simulink model "MPC_framework"  (Simulink 7.9)
settings: Solver=FixedStepDiscrete  StartTime=0.0  StopTime=10.0  FixedStep=0.01  RelTol=1e-3
PreLoadFcn:
  | RTWConfigurationCB('preloadfcn', bdroot);
InitFcn:
  | % START RTW CONFIGURATION CODE %
  | RTWConfigurationCB('rtw_target_initfcn',gcs);
  | % END RTW CONFIGURATION CODE %
libraries: mpc5xxobsoleteblocks x13, canblocks x12, simulink x2
settings Model: Creator=Bazs  LastModifiedBy=Bazs
settings OptimizationCC: InitFltsAndDblsToZero=on
settings DebuggingCC: SaveWithParameterizedLinksMsg=none  SignalResolutionControl=TryResolveAllWithWarning  MultiTaskDSMMsg=warning  MultiTaskCondExecSysMsg=none  FcnCallInpInsideContextMsg=Use local settings  StrictBusMsg=Warning
settings SFSimCC: SimParseCustomCode=off
settings RTWCC: IncludeERTFirstTime=on
settings GRTTargetCC: TargetFcnLib=ansi_tfl_tmw.mat  CombineOutputUpdateFcns=off  GRTInterface=on

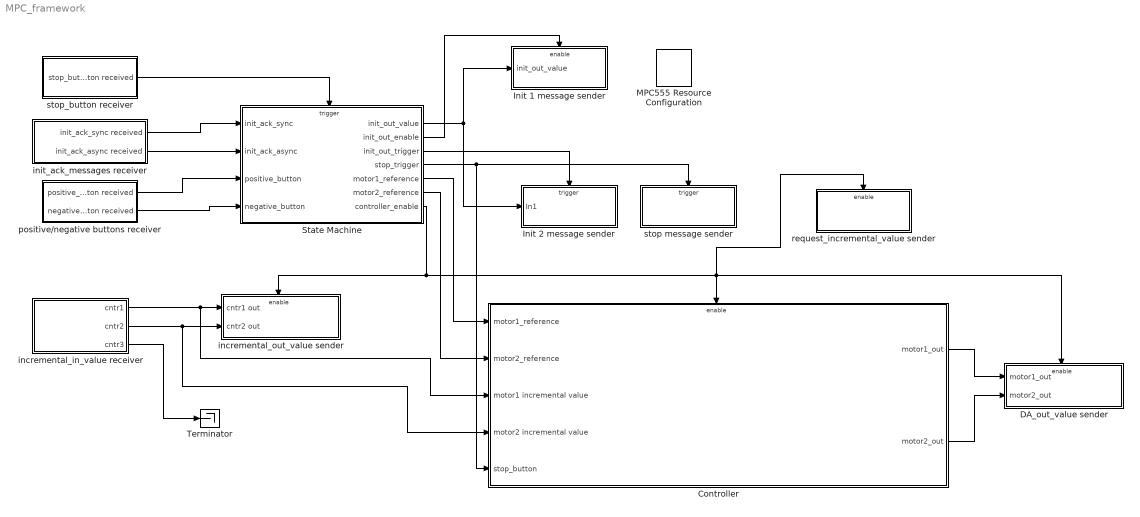
== system MPC_framework ==
  Controller : Subsystem
  DA_out_value sender : Subsystem  TreatAsAtomicUnit=on
  Init 1 message sender : Subsystem  TreatAsAtomicUnit=on
  Init 2 message sender : Subsystem  TreatAsAtomicUnit=on
  MPC555 Resource Configuration : mpc5xxobsoleteblocks/MPC555 Resource Configuration  Tag=RTW CONFIGURATION BLOCK  Priority=-100000  oldParentName=MPC_framework  oldBlockName=|
      | MPC_framework/MPC555
      | Resource
      | Configuration
  State Machine : Stateflow chart  TreatAsAtomicUnit=on
  Terminator : Terminator
  incremental_in_value receiver : Subsystem
  incremental_out_value sender : Subsystem  TreatAsAtomicUnit=on
  init_ack_messages receiver : Subsystem
  positive/negative buttons receiver : Subsystem
  request_incremental_value sender : Subsystem  TreatAsAtomicUnit=on
  stop message sender : Subsystem  TreatAsAtomicUnit=on
  stop_button receiver : Subsystem
  wires:
  State Machine/1(init_out_value) -> Init 1 message sender/1(init_out_value), Init 2 message sender/1(In1)
  State Machine/2(init_out_enable) -> Init 1 message sender/Enable
  init_ack_messages receiver/1(init_ack_sync received) -> State Machine/1(init_ack_sync)
  init_ack_messages receiver/2(init_ack_async received) -> State Machine/2(init_ack_async)
  State Machine/3(init_out_trigger) -> Init 2 message sender/Trigger
  stop_button receiver/1(stop_button received) -> State Machine/Trigger
  State Machine/4(stop_trigger) -> stop message sender/Trigger, Controller/5(stop_button)
  positive/negative buttons receiver/1(positive_button received) -> State Machine/3(positive_button)
  positive/negative buttons receiver/2(negative_button received) -> State Machine/4(negative_button)
  State Machine/7(controller_enable) -> Controller/Enable, DA_out_value sender/Enable, request_incremental_value sender/Enable, incremental_out_value sender/Enable
  State Machine/5(motor1_reference) -> Controller/1(motor1_reference)
  State Machine/6(motor2_reference) -> Controller/2(motor2_reference)
  Controller/1(motor1_out) -> DA_out_value sender/1(motor1_out)
  Controller/2(motor2_out) -> DA_out_value sender/2(motor2_out)
  incremental_in_value receiver/1(cntr1) -> incremental_out_value sender/1(cntr1 out), Controller/3(motor1 incremental value)
  incremental_in_value receiver/2(cntr2) -> incremental_out_value sender/2(cntr2 out), Controller/4(motor2 incremental value)
  incremental_in_value receiver/3(cntr3) -> Terminator/1

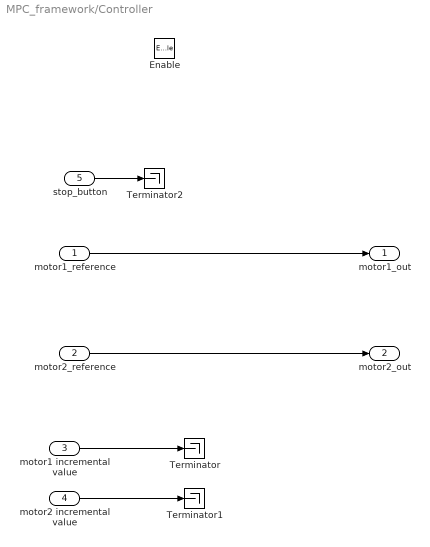
== system MPC_framework/Controller ==
  motor1_reference : Inport
  motor2_reference : Inport  Port=2
  motor1 incremental value : Inport  Port=3
  motor2 incremental value : Inport  Port=4
  stop_button : Inport  Port=5
  Enable : EnablePort
  Terminator : Terminator
  Terminator1 : Terminator
  Terminator2 : Terminator
  motor1_out : Outport
  motor2_out : Outport  Port=2
  wires:
  motor1 incremental value/1 -> Terminator/1
  motor2 incremental value/1 -> Terminator1/1
  motor1_reference/1 -> motor1_out/1
  motor2_reference/1 -> motor2_out/1
  stop_button/1 -> Terminator2/1

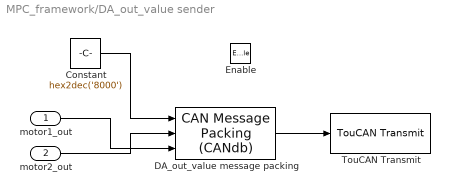
== system MPC_framework/DA_out_value sender ==
  motor1_out : Inport
  motor2_out : Inport  Port=2
  Enable : EnablePort
  Constant : Constant  Value=hex2dec('8000')
  DA_out_value message packing : canblocks/CAN Message Packing (CANdb)
  TouCAN Transmit : mpc5xxobsoleteblocks/CAN 2.0B Controller Module/TouCAN Transmit  module=A  tx_mode=Queued transmission with shared buffer  fifo_queue_length=8  bufferids=0  buffers_used=0, 1, 2  t=-1  enablePassThru=off
  wires:
  DA_out_value message packing/1 -> TouCAN Transmit/1
  motor1_out/1 -> DA_out_value message packing/3
  motor2_out/1 -> DA_out_value message packing/2
  Constant/1 -> DA_out_value message packing/1

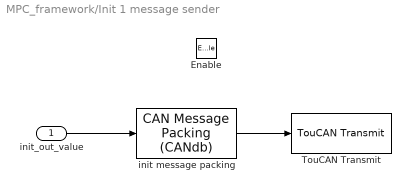
== system MPC_framework/Init 1 message sender ==
  init_out_value : Inport
  Enable : EnablePort
  TouCAN Transmit : mpc5xxobsoleteblocks/CAN 2.0B Controller Module/TouCAN Transmit  module=A  tx_mode=Queued transmission with shared buffer  fifo_queue_length=8  bufferids=0  buffers_used=0, 1, 2  t=-1  enablePassThru=off
  init message packing : canblocks/CAN Message Packing (CANdb)
  wires:
  init_out_value/1 -> init message packing/1
  init message packing/1 -> TouCAN Transmit/1

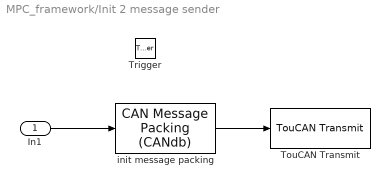
== system MPC_framework/Init 2 message sender ==
  In1 : Inport
  Trigger : TriggerPort
  TouCAN Transmit : mpc5xxobsoleteblocks/CAN 2.0B Controller Module/TouCAN Transmit  module=A  tx_mode=Queued transmission with shared buffer  fifo_queue_length=8  bufferids=0  buffers_used=0, 1, 2  t=-1  enablePassThru=off
  init message packing : canblocks/CAN Message Packing (CANdb)
  wires:
  In1/1 -> init message packing/1
  init message packing/1 -> TouCAN Transmit/1

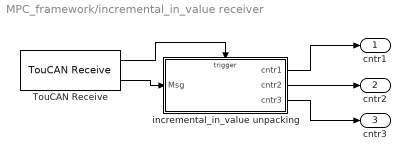
== system MPC_framework/incremental_in_value receiver ==
  TouCAN Receive : mpc5xxobsoleteblocks/CAN 2.0B Controller Module/TouCAN Receive  module=A  ids=hex2dec('07')  message_type=Standard (11-bit identifier)  notification_type=Function Call Outport  auto_select_buffer=on  bufferids=3  use_queue=off  queue_length=3  can_msg=Use unpacking block  t=-1
  incremental_in_value unpacking : Subsystem  TreatAsAtomicUnit=on
      settings: OpenFcn=open_system(gcb, 'force');
      mask Type: CAN Message Unpacking (CANdb)
      mask Description: CAN Message Unpacking (CANdb) Function-Call Subsystem Template
      mask Help: helpview([docroot '/toolbox/can_blocks/can_blocks.map'], 'template_CANdb_msg_unpack');
  cntr1 : Outport
  cntr2 : Outport  Port=2
  cntr3 : Outport  Port=3
  wires:
  incremental_in_value unpacking/1(cntr1) -> cntr1/1
  TouCAN Receive/2 -> incremental_in_value unpacking/1(Msg)
  TouCAN Receive/1 -> incremental_in_value unpacking/Trigger
  incremental_in_value unpacking/2(cntr2) -> cntr2/1
  incremental_in_value unpacking/3(cntr3) -> cntr3/1

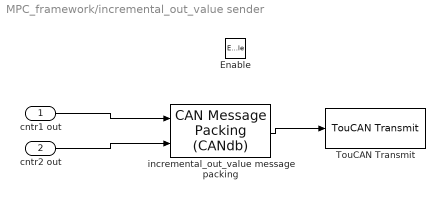
== system MPC_framework/incremental_out_value sender ==
  cntr1 out : Inport
  cntr2 out : Inport  Port=2
  Enable : EnablePort
  TouCAN Transmit : mpc5xxobsoleteblocks/CAN 2.0B Controller Module/TouCAN Transmit  module=A  tx_mode=Queued transmission with shared buffer  fifo_queue_length=8  bufferids=0  buffers_used=0, 1, 2  t=-1  enablePassThru=off
  incremental_out_value message packing : canblocks/CAN Message Packing (CANdb)
  wires:
  incremental_out_value message packing/1 -> TouCAN Transmit/1
  cntr1 out/1 -> incremental_out_value message packing/1
  cntr2 out/1 -> incremental_out_value message packing/2

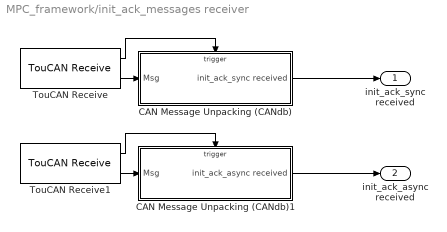
== system MPC_framework/init_ack_messages receiver ==
  CAN Message Unpacking (CANdb) : Subsystem  TreatAsAtomicUnit=on
      settings: OpenFcn=open_system(gcb, 'force');
      mask Type: CAN Message Unpacking (CANdb)
      mask Description: CAN Message Unpacking (CANdb) Function-Call Subsystem Template
      mask Help: helpview([docroot '/toolbox/can_blocks/can_blocks.map'], 'template_CANdb_msg_unpack');
  CAN Message Unpacking (CANdb)1 : Subsystem  TreatAsAtomicUnit=on
      settings: OpenFcn=open_system(gcb, 'force');
      mask Type: CAN Message Unpacking (CANdb)
      mask Description: CAN Message Unpacking (CANdb) Function-Call Subsystem Template
      mask Help: helpview([docroot '/toolbox/can_blocks/can_blocks.map'], 'template_CANdb_msg_unpack');
  TouCAN Receive : mpc5xxobsoleteblocks/CAN 2.0B Controller Module/TouCAN Receive  module=A  ids=hex2dec('02')  message_type=Standard (11-bit identifier)  notification_type=Function Call Outport  auto_select_buffer=on  bufferids=4  use_queue=off  queue_length=3  can_msg=Use unpacking block  t=-1
  TouCAN Receive1 : mpc5xxobsoleteblocks/CAN 2.0B Controller Module/TouCAN Receive  module=A  ids=hex2dec('03')  message_type=Standard (11-bit identifier)  notification_type=Function Call Outport  auto_select_buffer=on  bufferids=5  use_queue=off  queue_length=3  can_msg=Use unpacking block  t=-1
  init_ack_sync received : Outport
  init_ack_async received : Outport  Port=2
  wires:
  TouCAN Receive/1 -> CAN Message Unpacking (CANdb)/Trigger
  TouCAN Receive/2 -> CAN Message Unpacking (CANdb)/1(Msg)
  CAN Message Unpacking (CANdb)/1(init_ack_sync received) -> init_ack_sync received/1
  TouCAN Receive1/1 -> CAN Message Unpacking (CANdb)1/Trigger
  TouCAN Receive1/2 -> CAN Message Unpacking (CANdb)1/1(Msg)
  CAN Message Unpacking (CANdb)1/1(init_ack_async received) -> init_ack_async received/1

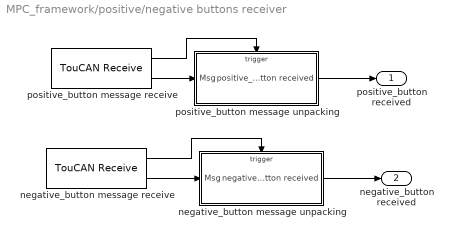
== system MPC_framework/positive/negative buttons receiver ==
  negative_button message receive : mpc5xxobsoleteblocks/CAN 2.0B Controller Module/TouCAN Receive  module=A  ids=hex2dec('09')  message_type=Standard (11-bit identifier)  notification_type=Function Call Outport  auto_select_buffer=on  bufferids=6  use_queue=off  queue_length=3  can_msg=Use unpacking block  t=-1
  negative_button message unpacking : Subsystem  TreatAsAtomicUnit=on
      settings: OpenFcn=open_system(gcb, 'force');
      mask Type: CAN Message Unpacking (CANdb)
      mask Description: CAN Message Unpacking (CANdb) Function-Call Subsystem Template
      mask Help: helpview([docroot '/toolbox/can_blocks/can_blocks.map'], 'template_CANdb_msg_unpack');
  positive_button message receive : mpc5xxobsoleteblocks/CAN 2.0B Controller Module/TouCAN Receive  module=A  ids=hex2dec('08')  message_type=Standard (11-bit identifier)  notification_type=Function Call Outport  auto_select_buffer=on  bufferids=7  use_queue=off  queue_length=3  can_msg=Use unpacking block  t=-1
  positive_button message unpacking : Subsystem  TreatAsAtomicUnit=on
      settings: OpenFcn=open_system(gcb, 'force');
      mask Type: CAN Message Unpacking (CANdb)
      mask Description: CAN Message Unpacking (CANdb) Function-Call Subsystem Template
      mask Help: helpview([docroot '/toolbox/can_blocks/can_blocks.map'], 'template_CANdb_msg_unpack');
  positive_button received : Outport
  negative_button received : Outport  Port=2
  wires:
  positive_button message unpacking/1(positive_button received) -> positive_button received/1
  positive_button message receive/2 -> positive_button message unpacking/1(Msg)
  positive_button message receive/1 -> positive_button message unpacking/Trigger
  negative_button message unpacking/1(negative_button received) -> negative_button received/1
  negative_button message receive/2 -> negative_button message unpacking/1(Msg)
  negative_button message receive/1 -> negative_button message unpacking/Trigger

== system MPC_framework/request_incremental_value sender ==
  Enable : EnablePort
  Constant : Constant  OutDataTypeStr=uint8  SampleTime=0.1
  TouCAN Transmit : mpc5xxobsoleteblocks/CAN 2.0B Controller Module/TouCAN Transmit  module=A  tx_mode=Queued transmission with shared buffer  fifo_queue_length=8  bufferids=0  buffers_used=0, 1, 2  t=-1  enablePassThru=off
  request_incremental_value message packing : canblocks/CAN Message Packing (CANdb)
  wires:
  Constant/1 -> request_incremental_value message packing/1
  request_incremental_value message packing/1 -> TouCAN Transmit/1

== system MPC_framework/stop message sender ==
  Trigger : TriggerPort
  Constant : Constant  OutDataTypeStr=uint8
  TouCAN Transmit : mpc5xxobsoleteblocks/CAN 2.0B Controller Module/TouCAN Transmit  module=A  tx_mode=Queued transmission with shared buffer  fifo_queue_length=8  bufferids=0  buffers_used=0, 1, 2  t=-1  enablePassThru=off
  stop message packing : canblocks/CAN Message Packing (CANdb)
  wires:
  stop message packing/1 -> TouCAN Transmit/1
  Constant/1 -> stop message packing/1

== system MPC_framework/stop_button receiver ==
  TouCAN Receive : mpc5xxobsoleteblocks/CAN 2.0B Controller Module/TouCAN Receive  module=A  ids=hex2dec('04')  message_type=Standard (11-bit identifier)  notification_type=Function Call Outport  auto_select_buffer=on  bufferids=8  use_queue=off  queue_length=3  can_msg=Use unpacking block  t=-1
  stop_button message packing : Subsystem  TreatAsAtomicUnit=on
      settings: OpenFcn=open_system(gcb, 'force');
      mask Type: CAN Message Unpacking (CANdb)
      mask Description: CAN Message Unpacking (CANdb) Function-Call Subsystem Template
      mask Help: helpview([docroot '/toolbox/can_blocks/can_blocks.map'], 'template_CANdb_msg_unpack');
  stop_button received : Outport
  wires:
  TouCAN Receive/1 -> stop_button message packing/Trigger
  TouCAN Receive/2 -> stop_button message packing/1(Msg)
  stop_button message packing/1(stop_button received) -> stop_button received/1

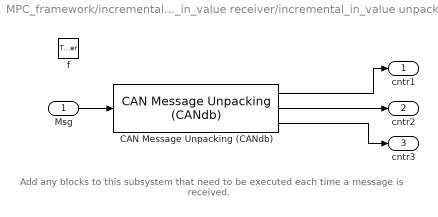
== system MPC_framework/incremental_in_value receiver/incremental_in_value unpacking ==
  note: Add any blocks to this subsystem that need to be
      | executed each time a message is received.
  Msg : Inport
  f : TriggerPort  TriggerType=function-call
  CAN Message Unpacking (CANdb) : canblocks/CAN Message Unpacking (CANdb)/CAN Message Unpacking (CANdb)
  cntr1 : Outport
  cntr2 : Outport  Port=2
  cntr3 : Outport  Port=3
  wires:
  CAN Message Unpacking (CANdb)/1 -> cntr1/1
  Msg/1 -> CAN Message Unpacking (CANdb)/1
  CAN Message Unpacking (CANdb)/2 -> cntr2/1
  CAN Message Unpacking (CANdb)/3 -> cntr3/1

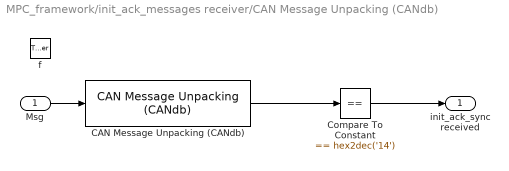
== system MPC_framework/init_ack_messages receiver/CAN Message Unpacking (CANdb) ==
  Msg : Inport
  f : TriggerPort  TriggerType=function-call
  CAN Message Unpacking (CANdb) : canblocks/CAN Message Unpacking (CANdb)/CAN Message Unpacking (CANdb)
  Compare To Constant : simulink/Logic and Bit Operations/Compare To Constant  relop===  const=hex2dec('14')  OutDataTypeStr=uint8  ZeroCross=off
  init_ack_sync received : Outport
  wires:
  Msg/1 -> CAN Message Unpacking (CANdb)/1
  CAN Message Unpacking (CANdb)/1 -> Compare To Constant/1
  Compare To Constant/1 -> init_ack_sync received/1

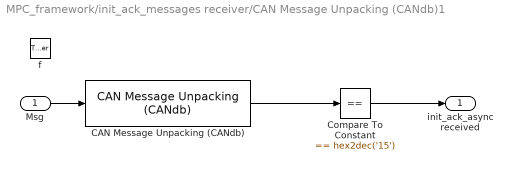
== system MPC_framework/init_ack_messages receiver/CAN Message Unpacking (CANdb)1 ==
  Msg : Inport
  f : TriggerPort  TriggerType=function-call
  CAN Message Unpacking (CANdb) : canblocks/CAN Message Unpacking (CANdb)/CAN Message Unpacking (CANdb)
  Compare To Constant : simulink/Logic and Bit Operations/Compare To Constant  relop===  const=hex2dec('15')  OutDataTypeStr=uint8  ZeroCross=off
  init_ack_async received : Outport
  wires:
  Compare To Constant/1 -> init_ack_async received/1
  CAN Message Unpacking (CANdb)/1 -> Compare To Constant/1
  Msg/1 -> CAN Message Unpacking (CANdb)/1

== system MPC_framework/positive/negative buttons receiver/negative_button message unpacking ==
  note: Add any blocks to this subsystem that need to be
      | executed each time a message is received.
  Msg : Inport
  f : TriggerPort  TriggerType=function-call
  CAN Message Unpacking (CANdb) : canblocks/CAN Message Unpacking (CANdb)/CAN Message Unpacking (CANdb)
  negative_button received : Outport
  wires:
  Msg/1 -> CAN Message Unpacking (CANdb)/1
  CAN Message Unpacking (CANdb)/1 -> negative_button received/1

== system MPC_framework/positive/negative buttons receiver/positive_button message unpacking ==
  note: Add any blocks to this subsystem that need to be
      | executed each time a message is received.
  Msg : Inport
  f : TriggerPort  TriggerType=function-call
  CAN Message Unpacking (CANdb) : canblocks/CAN Message Unpacking (CANdb)/CAN Message Unpacking (CANdb)
  positive_button received : Outport
  wires:
  CAN Message Unpacking (CANdb)/1 -> positive_button received/1
  Msg/1 -> CAN Message Unpacking (CANdb)/1

== system MPC_framework/stop_button receiver/stop_button message packing ==
  note: Add any blocks to this subsystem that need to be
      | executed each time a message is received.
  Msg : Inport
  f : TriggerPort  TriggerType=function-call
  CAN Message Unpacking (CANdb) : canblocks/CAN Message Unpacking (CANdb)/CAN Message Unpacking (CANdb)
  stop_button received : Outport
  wires:
  Msg/1 -> CAN Message Unpacking (CANdb)/1
  CAN Message Unpacking (CANdb)/1 -> stop_button received/1

== stateflow chart State Machine ==
  settings: executeAtInitialization=1
  state INIT
    entry: init_out_value=1;
    init_out_enable=1;
  state INIT_ACK
    entry: init_out_enable=0;
    init_out_value=2;
    init_out_trigger=1;
  state OPERATION
    during: controller_enable=1;
    state MOVING
      state POSITIVE_MOVEMENT
        entry: motor1_reference=motor_positive_value;
      state NEGATIVE_MOVEMENT
        entry: motor1_reference=motor_negative_value;
    state STOPPED
      entry: motor1_reference=motor_stopped_value;
      motor2_reference=motor_stopped_value;
      exit: stop_trigger=0;
    (default) -> STOPPED
    MOVING -> STOPPED [order 1] : stop_button/stop_trigger=1;
    STOPPED -> POSITIVE_MOVEMENT [order 1] : [positive_button==1]
    STOPPED -> NEGATIVE_MOVEMENT [order 2] : [negative_button==1]
    MOVING -> STOPPED [order 3] : [positive_button==2]
    MOVING -> STOPPED [order 2] : [negative_button==2]
  (default) -> INIT
  INIT -> INIT_ACK : [init_ack_sync==1 && init_ack_async==1]
  INIT_ACK -> OPERATION
  data: motor_positive_value constant double =hex2dec('A000'); motor_negative_value constant double =hex2dec('6000'); init_out_value output uint8 =0; init_out_enable output uint8 =0; init_ack_sync input uint8; init_ack_async input uint8; init_out_trigger output uint8 =0; stop_trigger output uint8 =0; positive_button input uint8 =0; negative_button input uint8; motor1_reference output uint16 =hex2dec('8000'); motor2_reference output uint16 =hex2dec('8000'); motor_stopped_value constant double =hex2dec('8000'); controller_enable output uint8 =0
  events: stop_button input RISING_EDGE_EVENT
